simulink model "Martin_fuzzy_chemo_faisal_fecsc21_weight_sajal_ver2"  (R2020a)
settings: Solver=VariableStepAuto  StartTime=0.0  StopTime=120  RelTol=1e-5  EnableMultiTasking=on
libraries: fuzblock x2, dspsigops x1
settings Model: Creator=nadia  LastModifiedBy=Hp
settings DataIOCC: LimitDataPoints=on  SaveFormat=Array  SignalLoggingSaveFormat=ModelDataLogs  ReturnWorkspaceOutputs=off
settings OptimizationCC: ExpressionDepthLimit=2147483647  LifeSpan=inf
settings DebuggingCC: UnderspecifiedInitializationDetection=Classic  MergeDetectMultiDrivingBlocksExec=none  SolverPrmCheckMsg=warning  FcnCallInpInsideContextMsg=warning  StateNameClashWarn=warning  SFUnexpectedBacktrackingDiag=warning  SFNoUnconditionalDefaultTransitionDiag=warning  SFExecutionAtInitializationDiag=none  ArithmeticOperatorsInVariantConditions=warning
settings HardwareCC: ProdBitPerPointer=32  ProdBitPerSizeT=32  ProdBitPerPtrDiffT=32  ProdLargestAtomicFloat=None  ProdIntDivRoundTo=Undefined  ProdEndianess=Unspecified  ProdWordSize=32  ProdHWDeviceType=32-bit Generic
settings ModelReferenceCC: PropagateSignalLabelsOutOfModel=off
settings SFSimCC: SimUseLocalCustomCode=off  SimParseCustomCode=off  CustomCodeUndefinedFunction=UseInterfaceOnly
settings RTWCC: RTWUseLocalCustomCode=off
settings CodeAppCC: StateflowObjectComments=on
settings GRTTargetCC: TargetLangStandard=C89/C90 (ANSI)  CombineOutputUpdateFcns=off  GRTInterface=on
settings ConfigComp: CovMetricSettings=dw  CovHtmlReporting=on  CovSaveCumulativeToWorkspaceVar=on  CovSaveSingleToWorkspaceVar=on  CovExternalEMLEnable=off

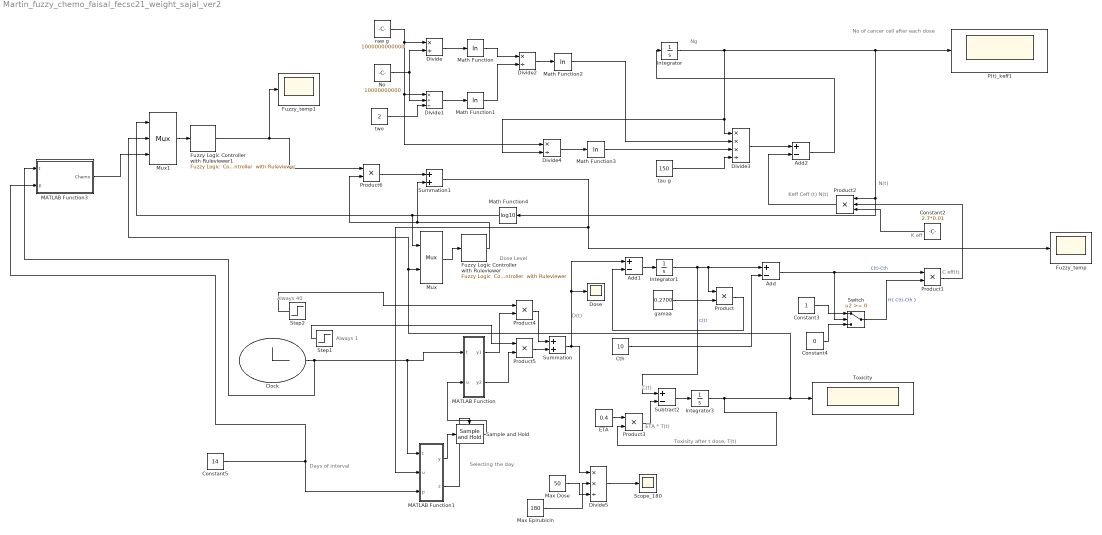
== system Martin_fuzzy_chemo_faisal_fecsc21_weight_sajal_ver2 ==
  note: Always 40
  note: Selecting the day
  note: Dose Level
  note: Days of interval
  note: D(t)
  note: ETA * T(t)
  note: C(t)
  note: Toxisity after t dose, T(t)
  note: N(t)
  note: No of cancer cell after each dose
  note: K eff
  note: Keff Ceff (t) N(t)
  note: C eff(t)
  note: Ng
  note: Always 1
  Add : Sum  Inputs=+-
  Add1 : Sum  Inputs=+-
  Add2 : Sum  Inputs=+-
  Clock : Clock
      settings: Decimation=120
  Constant2 : Constant  Value=2.7*0.01
  Constant3 : Constant
  Constant4 : Constant  Value=0
  Constant5 : Constant  Value=14
  Cth : Constant  Value=10
  Divide : Product  Inputs=*/
  Divide1 : Product  Inputs=*//
  Divide2 : Product  Inputs=*/
  Divide3 : Product  Inputs=***/
  Divide4 : Product  Inputs=*/
  Divide5 : Product  Inputs=**/
  Dose : Scope
  ETA : Constant  Value=0.4
  Fuzzy Logic Controller with Ruleviewer : fuzblock/Fuzzy Logic  Controller  with Ruleviewer  fismatrix=FES_1_gaussian_TTD_2  Ts=2
  Fuzzy Logic Controller with Ruleviewer1 : fuzblock/Fuzzy Logic  Controller  with Ruleviewer  fismatrix=FES2_ver7_TTC_3  Ts=2
  Fuzzy_temp : Scope
  Fuzzy_temp1 : Scope
  Integrator : Integrator  InitialCondition=10000000000  IgnoreLimit=on
  Integrator1 : Integrator
  Integrator3 : Integrator
  MATLAB Function : MATLAB Function  TreatAsAtomicUnit=on
  MATLAB Function1 : MATLAB Function  TreatAsAtomicUnit=on
  MATLAB Function3 : MATLAB Function  TreatAsAtomicUnit=on
  Math Function{,1..3} (4 alike) : Math  Operator=log  SignedPower=on  SaturateOnIntegerOverflow=on
  Math Function4 : Math  Operator=log10  SignedPower=on  SaturateOnIntegerOverflow=on
  Max Dose : Constant  Value=50
  Max Epirubicin : Constant  Value=180
  Mux : Mux  Inputs=2
      settings: DisplayOption=signals
  Mux1 : Mux  Inputs=3
      settings: DisplayOption=signals
  No : Constant  Value=10000000000
  P(t)_keff1 : Scope
  Product{,1,3..6} (6 alike) : Product  RndMeth=Zero
  Product2 : Product  Inputs=3  RndMeth=Zero
  Sample and Hold : dspsigops/Sample and Hold  trig=Rising edge  initCond=0  latchinput=off
  Scope_180 : Scope
  Step1 : Step  Time=0  SampleTime=0
  Step2 : Step  Time=0  After=40  SampleTime=0
  Subtract2 : Sum  Inputs=+-
  Summation : Sum
  Summation1 : Sum
  Switch : Switch  ZeroCross=off
  Toxicity : Scope
  gamaa : Constant  Value=0.2700
  raw g : Constant  Value=1000000000000
  tau g : Constant  Value=150
  two : Constant  Value=2
  wires:
  raw g/1 -> Divide/1, Divide1/1, Divide4/1
  No/1 -> Divide/2, Divide1/2
  Divide/1 -> Math Function/1
  Divide1/1 -> Math Function1/1
  Math Function/1 -> Divide2/1
  Math Function1/1 -> Divide2/2
  Divide2/1 -> Math Function2/1
  Divide4/1 -> Math Function3/1
  tau g/1 -> Divide3/4
  Math Function3/1 -> Divide3/3
  Math Function2/1 -> Divide3/2
  Integrator/1 -> Divide3/1, Divide4/2, P(t)_keff1/1, Product2/1, Math Function4/1
  two/1 -> Divide1/3
  Add1/1 -> Integrator1/1
  Integrator1/1 -> Subtract2/1, Product/1, Add/1  "C(t)"
  gamaa/1 -> Product/2
  Product/1 -> Add1/2
  Cth/1 -> Add/2
  Add/1 -> Product1/1, Switch/2  "C(t)-Cth"
  Constant3/1 -> Switch/1
  Constant4/1 -> Switch/3
  Switch/1 -> Product1/2  "H{ C(t)-Cth }"
  Product1/1 -> Product2/2
  Constant2/1 -> Product2/3
  Product2/1 -> Add2/2
  Divide3/1 -> Add2/1
  Add2/1 -> Integrator/1
  Product3/1 -> Subtract2/2
  ETA/1 -> Product3/1
  Subtract2/1 -> Integrator3/1
  Product4/1 -> Summation/1
  Mux/1 -> Fuzzy Logic Controller with Ruleviewer/1
  Clock/1 -> MATLAB Function3/1(t), MATLAB Function/1(t), MATLAB Function1/1(t)
  Product5/1 -> Summation/2
  Summation/1 -> Divide5/1, Dose/1, Add1/1
  MATLAB Function/1(y1) -> Product4/2
  Fuzzy Logic Controller with Ruleviewer/1 -> Summation1/2, Product6/2
  MATLAB Function1/1(y) -> Sample and Hold/1
  Step1/1 -> Product5/1
  MATLAB Function/2(y2) -> Product5/2
  Sample and Hold/1 -> MATLAB Function/2(u)
  MATLAB Function1/2(z) -> Sample and Hold/Trigger
  Math Function4/1 -> Mux1/1, Mux/1
  Constant5/1 -> MATLAB Function3/2(p), MATLAB Function1/3(p)
  Step2/1 -> Product4/1
  Integrator3/1 -> Product3/2, Mux1/2, Mux/2, Toxicity/1
  Mux1/1 -> Fuzzy Logic Controller with Ruleviewer1/1
  MATLAB Function3/1(Chemo) -> Mux1/3
  Fuzzy Logic Controller with Ruleviewer1/1 -> Fuzzy_temp1/1, Product6/1
  Product6/1 -> Summation1/1
  Summation1/1 -> Fuzzy_temp/1, MATLAB Function1/2(u)
  Divide5/1 -> Scope_180/1
  Max Dose/1 -> Divide5/3
  Max Epirubicin/1 -> Divide5/2

== matlab function Martin_fuzzy_chemo_faisal_fecsc21_weight_sajal_ver2/MATLAB Function1 ==
  data: t input; u input; y output; z output; p input
function [y,z] = fcn1(t,u,p)
%#codegen

disp(t)

z=0;
if t>3 && mod((t-1),p)==0
    y=u; 
     z=1;
elseif mod((t-3),p)==0
    y=0;
    z=1;
elseif t==1
    y=u;
    z=1;
else
    y=0;
end
if t==2
    y=0;
    z=1;
end
end

== matlab function Martin_fuzzy_chemo_faisal_fecsc21_weight_sajal_ver2/MATLAB Function ==
  data: t input; u input; y1 output; y2 output
function [y1,y2] = drug_scheduling(t,u)


%#codegen
y1=0;
y2=0;
%temp=0;
if (t>=0)&& (t<=364)
     y1=0; 
     y2=u;
 else
     y1=0; 
     y2=0;
 end
end

== matlab function Martin_fuzzy_chemo_faisal_fecsc21_weight_sajal_ver2/MATLAB Function3 ==
  data: t input; Chemo output; p input
function Chemo  = fcn1(t,p)  %t--.each day ,P-->interval time, u--> dose amount

Weight_14_120_inc = [90,90,0,0,0,0,0,0,0,0,0,0,0,0,97,97,97,97,0,0,0,0,0,0,0,0,0,0,104,104,104,104,0,0,0,0,0,0,0,0,0,0,111,111,111,111,0,0,0,0,0,0,0,0,0,0,118,118,118,118,0,0,0,0,0,0,0,0,0,0,125,125,125,125,0,0,0,0,0,0,0,0,0,0,132,132,132,132,0,0,0,0,0,0,0,0,0,0,139,139,139,139,0,0,0,0,0,0,0,0,0,0,146,146,146,146,0,0,0,0,0];
% Weight_14_120_dec = [110,110,110,0,0,0,0,0,0,0,0,0,0,0,104,104,104,104,0,0,0,0,0,0,0,0,0,0,98,98,98,98,0,0,0,0,0,0,0,0,0,0,92,92,92,92,0,0,0,0,0,0,0,0,0,0,86,86,86,86,0,0,0,0,0,0,0,0,0,0,80,80,80,80,0,0,0,0,0,0,0,0,0,0,74,74,74,74,0,0,0,0,0,0,0,0,0,0,68,68,68,68,0,0,0,0,0,0,0,0,0,0,64,64,64,64,0,0,0,0,0];
% Weight_14_120_mix = [65,65,65,0,0,0,0,0,0,0,0,0,0,0,70,70,70,70,0,0,0,0,0,0,0,0,0,0,75,75,75,75,0,0,0,0,0,0,0,0,0,0,80,80,80,80,0,0,0,0,0,0,0,0,0,0,86,86,86,86,0,0,0,0,0,0,0,0,0,0,80,80,80,80,0,0,0,0,0,0,0,0,0,0,74,74,74,74,0,0,0,0,0,0,0,0,0,0,80,80,80,80,0,0,0,0,0,0,0,0,0,0,80,80,80,80,0,0,0,0,0];


if t<1
   Chemo=0; 
elseif (mod (t,1)==0)
    BSA= ((Weight_14_120_inc(t) * 4 ) + 7)/ (90 + Weight_14_120_inc(t));
    Chemo = BSA*100;
else 
    Chemo = 0;
end
end
